simulink model "stateFlowCalc"  (R2016b)
settings: Solver=FixedStepDiscrete  StartTime=0.0  StopTime=10.0  RelTol=1e-3
settings Model: Creator=Radwa  LastModifiedBy=Radwa
settings SolverCC: EnableConcurrentExecution=on
settings DataIOCC: ReturnWorkspaceOutputs=on
settings OptimizationCC: DefaultParameterBehavior=Inlined  EnhancedBackFolding=on  PassReuseOutputArgsAs=Individual arguments
settings DebuggingCC: ParameterTunabilityLossMsg=error
settings SFSimCC: SimUseLocalCustomCode=on
settings RTWCC: SystemTargetFile=ert.tlc  GenCodeOnly=on  TemplateMakefile=ert_default_tmf  Description=Embedded Coder  GenerateReport=on  RTWUseLocalCustomCode=on  IncludeHyperlinkInReport=on  LaunchReport=on  GenerateTraceInfo=on  GenerateTraceReport=on  GenerateTraceReportSl=on  GenerateTraceReportSf=on  GenerateTraceReportEml=on
settings CodeAppCC: ForceParamTrailComments=on  IgnoreCustomStorageClasses=off  OperatorAnnotations=on  SimulinkDataObjDesc=on  SFDataObjDesc=on  InsertBlockDesc=on
settings ERTTargetCC: TargetLangStandard=C99 (ISO)  MultiwordLength=256  GenerateSampleERTMain=on  InlinedParameterPlacement=NonHierarchical  ERTCustomFileTemplate=example_file_process.tlc

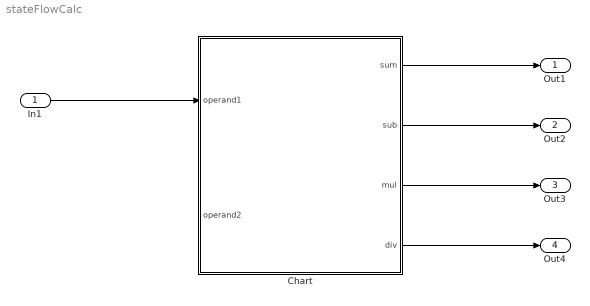
== system stateFlowCalc ==
  In1 : Inport
  Chart : Stateflow chart  TreatAsAtomicUnit=on
  Out1 : Outport
  Out2 : Outport  Port=2
  Out3 : Outport  Port=3
  Out4 : Outport  Port=4
  wires:
  In1/1 -> Chart/1(operand1)
  ? -> Chart/2(operand2)
  Chart/1(sum) -> Out1/1
  Chart/2(sub) -> Out2/1
  Chart/3(mul) -> Out3/1
  Chart/4(div) -> Out4/1

== stateflow chart stateFlowCalc/Chart ==
  state CalcState
    entry: sum=operand1+operand2;
    sub=operand1-operand2;
    mul=operand1*operand2;
  (default) -> state7
  state7 -> (junction 15)
  (junction 15) -> (junction 16) [order 1] : [operand2==0]
  (junction 15) -> (junction 17) [order 2] : {div=operand1/operand2;}
  (junction 16) -> (junction 18) : {div=0;}
  (junction 18) -> (junction 17)
  (junction 17) -> (junction 19)
  data: operand1 input; operand2 input; sum output; sub output; mul output; div output
